simulink model "untitled"  (R2021a)
settings: Solver=VariableStepAuto  StartTime=0.0  StopTime=5  FixedStep=0.01  MaxStep=0.0001  RelTol=1e-3
undefined symbols (not defined in the file or in its folder): fl
settings Model: Creator=umut  LastModifiedBy=umut

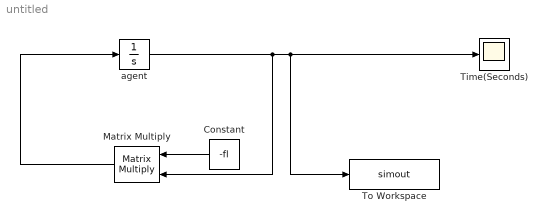
== system untitled ==
  Constant : Constant  Value=-fl
  Matrix Multiply : Product  Multiplication=Matrix(*)
  Time(Seconds) : Scope
      settings: AttributesFormatString=%<YLabel>
  To Workspace : ToWorkspace  VariableName=simout  SaveFormat=Timeseries  SampleTime=-1
  agent : Integrator  InitialCondition=[3;1;5;8;2]
  wires:
  agent/1 -> Matrix Multiply/2, To Workspace/1, Time(Seconds)/1
  Constant/1 -> Matrix Multiply/1
  Matrix Multiply/1 -> agent/1
